simulink model "c00003M_harness"  (R2018a)
settings: Solver=FixedStepAuto  StartTime=0.0  StopTime=300  FixedStep=0.1  RelTol=1e-3
undefined symbols (not defined in the file): A1, hmax, PriorityTank, R1, R2, sigbuilder_block
(part 5 of 44)

== system c00003M_harness/M022 ==
  note: VALUES
      | ---------------------------------
      | ControlType = 1 | 2 | 3
      | FillTank = 0 | 1
      | EmptyTank = 0 | 1
      | ManualReference between 0 and 1
      | Tempreature between 0 and 100
      | EmergencyButton = 0 | 1
      | LiquidLevel between 0 and 1 (hmax)
  note: Inputs For Tank2
  note: NAMES
      | --------------------------------------------
      | CT1 = ControlType Tank 1
      | F1 = Fill Tank 1
      | E1 = Empty Tank 1
      | MR1 = Manual Reference Tank1
      | T1 = Temperature Tank 1
      | EB1 = Emergency Button Tank 1
      | LL1 = Liquid Level 1
  note: Inputs For Tank3
  note: Inputs For Tank1
  CT1 : Inport
  F1 : Inport  Port=2
  E1 : Inport  Port=3
  MR1 : Inport  Port=4
  T1 : Inport  Port=5
  EB1 : Inport  Port=6
  CT2 : Inport  Port=7
  F2 : Inport  Port=8
  E2 : Inport  Port=9
  MR2 : Inport  Port=10
  T2 : Inport  Port=11
  EB2 : Inport  Port=12
  Tank1 : Subsystem
  Tank2 : Subsystem
  LL1 : Outport
  LL2 : Outport  Port=2
  wires:
  EB1/1 -> Tank1/6(EB1)
  Tank2/1(LL2) -> LL2/1, Tank1/7(LL2)
  EB2/1 -> Tank2/6(EB2)
  CT2/1 -> Tank2/1(CT2)
  MR1/1 -> Tank1/4(MR1)
  T1/1 -> Tank1/5(T1)
  Tank1/1(LL1) -> LL1/1, Tank2/7(LL1)
  F2/1 -> Tank2/2(F2)
  E2/1 -> Tank2/3(E2)
  F1/1 -> Tank1/2(F1)
  E1/1 -> Tank1/3(E1)
  T2/1 -> Tank2/5(T2)
  CT1/1 -> Tank1/1(CT1)
  MR2/1 -> Tank2/4(MR2)

== system c00003M_harness/M023 ==
  note: VALUES
      | ---------------------------------
      | ControlType = 1 | 2 | 3
      | FillTank = 0 | 1
      | EmptyTank = 0 | 1
      | ManualReference between 0 and 1
      | Tempreature between 0 and 100
      | EmergencyButton = 0 | 1
      | LiquidLevel between 0 and 1 (hmax)
  note: Inputs For Tank2
  note: NAMES
      | --------------------------------------------
      | CT1 = ControlType Tank 1
      | F1 = Fill Tank 1
      | E1 = Empty Tank 1
      | MR1 = Manual Reference Tank1
      | T1 = Temperature Tank 1
      | EB1 = Emergency Button Tank 1
      | LL1 = Liquid Level 1
  note: Inputs For Tank3
  note: Inputs For Tank1
  CT1 : Inport
  F1 : Inport  Port=2
  E1 : Inport  Port=3
  MR1 : Inport  Port=4
  T1 : Inport  Port=5
  EB1 : Inport  Port=6
  CT2 : Inport  Port=7
  F2 : Inport  Port=8
  E2 : Inport  Port=9
  MR2 : Inport  Port=10
  T2 : Inport  Port=11
  EB2 : Inport  Port=12
  Tank1 : Subsystem
  Tank2 : Subsystem
  LL1 : Outport
  LL2 : Outport  Port=2
  wires:
  EB1/1 -> Tank1/6(EB1)
  Tank2/1(LL2) -> LL2/1, Tank1/7(LL2)
  EB2/1 -> Tank2/6(EB2)
  CT2/1 -> Tank2/1(CT2)
  MR1/1 -> Tank1/4(MR1)
  T1/1 -> Tank1/5(T1)
  Tank1/1(LL1) -> LL1/1, Tank2/7(LL1)
  F2/1 -> Tank2/2(F2)
  E2/1 -> Tank2/3(E2)
  F1/1 -> Tank1/2(F1)
  E1/1 -> Tank1/3(E1)
  T2/1 -> Tank2/5(T2)
  CT1/1 -> Tank1/1(CT1)
  MR2/1 -> Tank2/4(MR2)

== system c00003M_harness/M024 ==
  note: VALUES
      | ---------------------------------
      | ControlType = 1 | 2 | 3
      | FillTank = 0 | 1
      | EmptyTank = 0 | 1
      | ManualReference between 0 and 1
      | Tempreature between 0 and 100
      | EmergencyButton = 0 | 1
      | LiquidLevel between 0 and 1 (hmax)
  note: Inputs For Tank2
  note: NAMES
      | --------------------------------------------
      | CT1 = ControlType Tank 1
      | F1 = Fill Tank 1
      | E1 = Empty Tank 1
      | MR1 = Manual Reference Tank1
      | T1 = Temperature Tank 1
      | EB1 = Emergency Button Tank 1
      | LL1 = Liquid Level 1
  note: Inputs For Tank3
  note: Inputs For Tank1
  CT1 : Inport
  F1 : Inport  Port=2
  E1 : Inport  Port=3
  MR1 : Inport  Port=4
  T1 : Inport  Port=5
  EB1 : Inport  Port=6
  CT2 : Inport  Port=7
  F2 : Inport  Port=8
  E2 : Inport  Port=9
  MR2 : Inport  Port=10
  T2 : Inport  Port=11
  EB2 : Inport  Port=12
  Tank1 : Subsystem
  Tank2 : Subsystem
  LL1 : Outport
  LL2 : Outport  Port=2
  wires:
  EB1/1 -> Tank1/6(EB1)
  Tank2/1(LL2) -> LL2/1, Tank1/7(LL2)
  EB2/1 -> Tank2/6(EB2)
  CT2/1 -> Tank2/1(CT2)
  MR1/1 -> Tank1/4(MR1)
  T1/1 -> Tank1/5(T1)
  Tank1/1(LL1) -> LL1/1, Tank2/7(LL1)
  F2/1 -> Tank2/2(F2)
  E2/1 -> Tank2/3(E2)
  F1/1 -> Tank1/2(F1)
  E1/1 -> Tank1/3(E1)
  T2/1 -> Tank2/5(T2)
  CT1/1 -> Tank1/1(CT1)
  MR2/1 -> Tank2/4(MR2)

== system c00003M_harness/M025 ==
  note: VALUES
      | ---------------------------------
      | ControlType = 1 | 2 | 3
      | FillTank = 0 | 1
      | EmptyTank = 0 | 1
      | ManualReference between 0 and 1
      | Tempreature between 0 and 100
      | EmergencyButton = 0 | 1
      | LiquidLevel between 0 and 1 (hmax)
  note: Inputs For Tank2
  note: NAMES
      | --------------------------------------------
      | CT1 = ControlType Tank 1
      | F1 = Fill Tank 1
      | E1 = Empty Tank 1
      | MR1 = Manual Reference Tank1
      | T1 = Temperature Tank 1
      | EB1 = Emergency Button Tank 1
      | LL1 = Liquid Level 1
  note: Inputs For Tank3
  note: Inputs For Tank1
  CT1 : Inport
  F1 : Inport  Port=2
  E1 : Inport  Port=3
  MR1 : Inport  Port=4
  T1 : Inport  Port=5
  EB1 : Inport  Port=6
  CT2 : Inport  Port=7
  F2 : Inport  Port=8
  E2 : Inport  Port=9
  MR2 : Inport  Port=10
  T2 : Inport  Port=11
  EB2 : Inport  Port=12
  Tank1 : Subsystem
  Tank2 : Subsystem
  LL1 : Outport
  LL2 : Outport  Port=2
  wires:
  EB1/1 -> Tank1/6(EB1)
  Tank2/1(LL2) -> LL2/1, Tank1/7(LL2)
  EB2/1 -> Tank2/6(EB2)
  CT2/1 -> Tank2/1(CT2)
  MR1/1 -> Tank1/4(MR1)
  T1/1 -> Tank1/5(T1)
  Tank1/1(LL1) -> LL1/1, Tank2/7(LL1)
  F2/1 -> Tank2/2(F2)
  E2/1 -> Tank2/3(E2)
  F1/1 -> Tank1/2(F1)
  E1/1 -> Tank1/3(E1)
  T2/1 -> Tank2/5(T2)
  CT1/1 -> Tank1/1(CT1)
  MR2/1 -> Tank2/4(MR2)

== system c00003M_harness/M026 ==
  note: VALUES
      | ---------------------------------
      | ControlType = 1 | 2 | 3
      | FillTank = 0 | 1
      | EmptyTank = 0 | 1
      | ManualReference between 0 and 1
      | Tempreature between 0 and 100
      | EmergencyButton = 0 | 1
      | LiquidLevel between 0 and 1 (hmax)
  note: Inputs For Tank2
  note: NAMES
      | --------------------------------------------
      | CT1 = ControlType Tank 1
      | F1 = Fill Tank 1
      | E1 = Empty Tank 1
      | MR1 = Manual Reference Tank1
      | T1 = Temperature Tank 1
      | EB1 = Emergency Button Tank 1
      | LL1 = Liquid Level 1
  note: Inputs For Tank3
  note: Inputs For Tank1
  CT1 : Inport
  F1 : Inport  Port=2
  E1 : Inport  Port=3
  MR1 : Inport  Port=4
  T1 : Inport  Port=5
  EB1 : Inport  Port=6
  CT2 : Inport  Port=7
  F2 : Inport  Port=8
  E2 : Inport  Port=9
  MR2 : Inport  Port=10
  T2 : Inport  Port=11
  EB2 : Inport  Port=12
  Tank1 : Subsystem
  Tank2 : Subsystem
  LL1 : Outport
  LL2 : Outport  Port=2
  wires:
  EB1/1 -> Tank1/6(EB1)
  Tank2/1(LL2) -> LL2/1, Tank1/7(LL2)
  EB2/1 -> Tank2/6(EB2)
  CT2/1 -> Tank2/1(CT2)
  MR1/1 -> Tank1/4(MR1)
  T1/1 -> Tank1/5(T1)
  Tank1/1(LL1) -> LL1/1, Tank2/7(LL1)
  F2/1 -> Tank2/2(F2)
  E2/1 -> Tank2/3(E2)
  F1/1 -> Tank1/2(F1)
  E1/1 -> Tank1/3(E1)
  T2/1 -> Tank2/5(T2)
  CT1/1 -> Tank1/1(CT1)
  MR2/1 -> Tank2/4(MR2)

== system c00003M_harness/M027 ==
  note: VALUES
      | ---------------------------------
      | ControlType = 1 | 2 | 3
      | FillTank = 0 | 1
      | EmptyTank = 0 | 1
      | ManualReference between 0 and 1
      | Tempreature between 0 and 100
      | EmergencyButton = 0 | 1
      | LiquidLevel between 0 and 1 (hmax)
  note: Inputs For Tank2
  note: NAMES
      | --------------------------------------------
      | CT1 = ControlType Tank 1
      | F1 = Fill Tank 1
      | E1 = Empty Tank 1
      | MR1 = Manual Reference Tank1
      | T1 = Temperature Tank 1
      | EB1 = Emergency Button Tank 1
      | LL1 = Liquid Level 1
  note: Inputs For Tank3
  note: Inputs For Tank1
  CT1 : Inport
  F1 : Inport  Port=2
  E1 : Inport  Port=3
  MR1 : Inport  Port=4
  T1 : Inport  Port=5
  EB1 : Inport  Port=6
  CT2 : Inport  Port=7
  F2 : Inport  Port=8
  E2 : Inport  Port=9
  MR2 : Inport  Port=10
  T2 : Inport  Port=11
  EB2 : Inport  Port=12
  Tank1 : Subsystem
  Tank2 : Subsystem
  LL1 : Outport
  LL2 : Outport  Port=2
  wires:
  EB1/1 -> Tank1/6(EB1)
  Tank2/1(LL2) -> LL2/1, Tank1/7(LL2)
  EB2/1 -> Tank2/6(EB2)
  CT2/1 -> Tank2/1(CT2)
  MR1/1 -> Tank1/4(MR1)
  T1/1 -> Tank1/5(T1)
  Tank1/1(LL1) -> LL1/1, Tank2/7(LL1)
  F2/1 -> Tank2/2(F2)
  E2/1 -> Tank2/3(E2)
  F1/1 -> Tank1/2(F1)
  E1/1 -> Tank1/3(E1)
  T2/1 -> Tank2/5(T2)
  CT1/1 -> Tank1/1(CT1)
  MR2/1 -> Tank2/4(MR2)

== system c00003M_harness/M028 ==
  note: VALUES
      | ---------------------------------
      | ControlType = 1 | 2 | 3
      | FillTank = 0 | 1
      | EmptyTank = 0 | 1
      | ManualReference between 0 and 1
      | Tempreature between 0 and 100
      | EmergencyButton = 0 | 1
      | LiquidLevel between 0 and 1 (hmax)
  note: Inputs For Tank2
  note: NAMES
      | --------------------------------------------
      | CT1 = ControlType Tank 1
      | F1 = Fill Tank 1
      | E1 = Empty Tank 1
      | MR1 = Manual Reference Tank1
      | T1 = Temperature Tank 1
      | EB1 = Emergency Button Tank 1
      | LL1 = Liquid Level 1
  note: Inputs For Tank3
  note: Inputs For Tank1
  CT1 : Inport
  F1 : Inport  Port=2
  E1 : Inport  Port=3
  MR1 : Inport  Port=4
  T1 : Inport  Port=5
  EB1 : Inport  Port=6
  CT2 : Inport  Port=7
  F2 : Inport  Port=8
  E2 : Inport  Port=9
  MR2 : Inport  Port=10
  T2 : Inport  Port=11
  EB2 : Inport  Port=12
  Tank1 : Subsystem
  Tank2 : Subsystem
  LL1 : Outport
  LL2 : Outport  Port=2
  wires:
  EB1/1 -> Tank1/6(EB1)
  Tank2/1(LL2) -> LL2/1, Tank1/7(LL2)
  EB2/1 -> Tank2/6(EB2)
  CT2/1 -> Tank2/1(CT2)
  MR1/1 -> Tank1/4(MR1)
  T1/1 -> Tank1/5(T1)
  Tank1/1(LL1) -> LL1/1, Tank2/7(LL1)
  F2/1 -> Tank2/2(F2)
  E2/1 -> Tank2/3(E2)
  F1/1 -> Tank1/2(F1)
  E1/1 -> Tank1/3(E1)
  T2/1 -> Tank2/5(T2)
  CT1/1 -> Tank1/1(CT1)
  MR2/1 -> Tank2/4(MR2)

== system c00003M_harness/M029 ==
  note: VALUES
      | ---------------------------------
      | ControlType = 1 | 2 | 3
      | FillTank = 0 | 1
      | EmptyTank = 0 | 1
      | ManualReference between 0 and 1
      | Tempreature between 0 and 100
      | EmergencyButton = 0 | 1
      | LiquidLevel between 0 and 1 (hmax)
  note: Inputs For Tank2
  note: NAMES
      | --------------------------------------------
      | CT1 = ControlType Tank 1
      | F1 = Fill Tank 1
      | E1 = Empty Tank 1
      | MR1 = Manual Reference Tank1
      | T1 = Temperature Tank 1
      | EB1 = Emergency Button Tank 1
      | LL1 = Liquid Level 1
  note: Inputs For Tank3
  note: Inputs For Tank1
  CT1 : Inport
  F1 : Inport  Port=2
  E1 : Inport  Port=3
  MR1 : Inport  Port=4
  T1 : Inport  Port=5
  EB1 : Inport  Port=6
  CT2 : Inport  Port=7
  F2 : Inport  Port=8
  E2 : Inport  Port=9
  MR2 : Inport  Port=10
  T2 : Inport  Port=11
  EB2 : Inport  Port=12
  Tank1 : Subsystem
  Tank2 : Subsystem
  LL1 : Outport
  LL2 : Outport  Port=2
  wires:
  EB1/1 -> Tank1/6(EB1)
  Tank2/1(LL2) -> LL2/1, Tank1/7(LL2)
  EB2/1 -> Tank2/6(EB2)
  CT2/1 -> Tank2/1(CT2)
  MR1/1 -> Tank1/4(MR1)
  T1/1 -> Tank1/5(T1)
  Tank1/1(LL1) -> LL1/1, Tank2/7(LL1)
  F2/1 -> Tank2/2(F2)
  E2/1 -> Tank2/3(E2)
  F1/1 -> Tank1/2(F1)
  E1/1 -> Tank1/3(E1)
  T2/1 -> Tank2/5(T2)
  CT1/1 -> Tank1/1(CT1)
  MR2/1 -> Tank2/4(MR2)

== system c00003M_harness/M030 ==
  note: VALUES
      | ---------------------------------
      | ControlType = 1 | 2 | 3
      | FillTank = 0 | 1
      | EmptyTank = 0 | 1
      | ManualReference between 0 and 1
      | Tempreature between 0 and 100
      | EmergencyButton = 0 | 1
      | LiquidLevel between 0 and 1 (hmax)
  note: Inputs For Tank2
  note: NAMES
      | --------------------------------------------
      | CT1 = ControlType Tank 1
      | F1 = Fill Tank 1
      | E1 = Empty Tank 1
      | MR1 = Manual Reference Tank1
      | T1 = Temperature Tank 1
      | EB1 = Emergency Button Tank 1
      | LL1 = Liquid Level 1
  note: Inputs For Tank3
  note: Inputs For Tank1
  CT1 : Inport
  F1 : Inport  Port=2
  E1 : Inport  Port=3
  MR1 : Inport  Port=4
  T1 : Inport  Port=5
  EB1 : Inport  Port=6
  CT2 : Inport  Port=7
  F2 : Inport  Port=8
  E2 : Inport  Port=9
  MR2 : Inport  Port=10
  T2 : Inport  Port=11
  EB2 : Inport  Port=12
  Tank1 : Subsystem
  Tank2 : Subsystem
  LL1 : Outport
  LL2 : Outport  Port=2
  wires:
  EB1/1 -> Tank1/6(EB1)
  Tank2/1(LL2) -> LL2/1, Tank1/7(LL2)
  EB2/1 -> Tank2/6(EB2)
  CT2/1 -> Tank2/1(CT2)
  MR1/1 -> Tank1/4(MR1)
  T1/1 -> Tank1/5(T1)
  Tank1/1(LL1) -> LL1/1, Tank2/7(LL1)
  F2/1 -> Tank2/2(F2)
  E2/1 -> Tank2/3(E2)
  F1/1 -> Tank1/2(F1)
  E1/1 -> Tank1/3(E1)
  T2/1 -> Tank2/5(T2)
  CT1/1 -> Tank1/1(CT1)
  MR2/1 -> Tank2/4(MR2)

== system c00003M_harness/M031 ==
  note: VALUES
      | ---------------------------------
      | ControlType = 1 | 2 | 3
      | FillTank = 0 | 1
      | EmptyTank = 0 | 1
      | ManualReference between 0 and 1
      | Tempreature between 0 and 100
      | EmergencyButton = 0 | 1
      | LiquidLevel between 0 and 1 (hmax)
  note: Inputs For Tank2
  note: NAMES
      | --------------------------------------------
      | CT1 = ControlType Tank 1
      | F1 = Fill Tank 1
      | E1 = Empty Tank 1
      | MR1 = Manual Reference Tank1
      | T1 = Temperature Tank 1
      | EB1 = Emergency Button Tank 1
      | LL1 = Liquid Level 1
  note: Inputs For Tank3
  note: Inputs For Tank1
  CT1 : Inport
  F1 : Inport  Port=2
  E1 : Inport  Port=3
  MR1 : Inport  Port=4
  T1 : Inport  Port=5
  EB1 : Inport  Port=6
  CT2 : Inport  Port=7
  F2 : Inport  Port=8
  E2 : Inport  Port=9
  MR2 : Inport  Port=10
  T2 : Inport  Port=11
  EB2 : Inport  Port=12
  Tank1 : Subsystem
  Tank2 : Subsystem
  LL1 : Outport
  LL2 : Outport  Port=2
  wires:
  EB1/1 -> Tank1/6(EB1)
  Tank2/1(LL2) -> LL2/1, Tank1/7(LL2)
  EB2/1 -> Tank2/6(EB2)
  CT2/1 -> Tank2/1(CT2)
  MR1/1 -> Tank1/4(MR1)
  T1/1 -> Tank1/5(T1)
  Tank1/1(LL1) -> LL1/1, Tank2/7(LL1)
  F2/1 -> Tank2/2(F2)
  E2/1 -> Tank2/3(E2)
  F1/1 -> Tank1/2(F1)
  E1/1 -> Tank1/3(E1)
  T2/1 -> Tank2/5(T2)
  CT1/1 -> Tank1/1(CT1)
  MR2/1 -> Tank2/4(MR2)

== system c00003M_harness/M032 ==
  note: VALUES
      | ---------------------------------
      | ControlType = 1 | 2 | 3
      | FillTank = 0 | 1
      | EmptyTank = 0 | 1
      | ManualReference between 0 and 1
      | Tempreature between 0 and 100
      | EmergencyButton = 0 | 1
      | LiquidLevel between 0 and 1 (hmax)
  note: Inputs For Tank2
  note: NAMES
      | --------------------------------------------
      | CT1 = ControlType Tank 1
      | F1 = Fill Tank 1
      | E1 = Empty Tank 1
      | MR1 = Manual Reference Tank1
      | T1 = Temperature Tank 1
      | EB1 = Emergency Button Tank 1
      | LL1 = Liquid Level 1
  note: Inputs For Tank3
  note: Inputs For Tank1
  CT1 : Inport
  F1 : Inport  Port=2
  E1 : Inport  Port=3
  MR1 : Inport  Port=4
  T1 : Inport  Port=5
  EB1 : Inport  Port=6
  CT2 : Inport  Port=7
  F2 : Inport  Port=8
  E2 : Inport  Port=9
  MR2 : Inport  Port=10
  T2 : Inport  Port=11
  EB2 : Inport  Port=12
  Tank1 : Subsystem
  Tank2 : Subsystem
  LL1 : Outport
  LL2 : Outport  Port=2
  wires:
  EB1/1 -> Tank1/6(EB1)
  Tank2/1(LL2) -> LL2/1, Tank1/7(LL2)
  EB2/1 -> Tank2/6(EB2)
  CT2/1 -> Tank2/1(CT2)
  MR1/1 -> Tank1/4(MR1)
  T1/1 -> Tank1/5(T1)
  Tank1/1(LL1) -> LL1/1, Tank2/7(LL1)
  F2/1 -> Tank2/2(F2)
  E2/1 -> Tank2/3(E2)
  F1/1 -> Tank1/2(F1)
  E1/1 -> Tank1/3(E1)
  T2/1 -> Tank2/5(T2)
  CT1/1 -> Tank1/1(CT1)
  MR2/1 -> Tank2/4(MR2)

== system c00003M_harness/M033 ==
  note: VALUES
      | ---------------------------------
      | ControlType = 1 | 2 | 3
      | FillTank = 0 | 1
      | EmptyTank = 0 | 1
      | ManualReference between 0 and 1
      | Tempreature between 0 and 100
      | EmergencyButton = 0 | 1
      | LiquidLevel between 0 and 1 (hmax)
  note: Inputs For Tank2
  note: NAMES
      | --------------------------------------------
      | CT1 = ControlType Tank 1
      | F1 = Fill Tank 1
      | E1 = Empty Tank 1
      | MR1 = Manual Reference Tank1
      | T1 = Temperature Tank 1
      | EB1 = Emergency Button Tank 1
      | LL1 = Liquid Level 1
  note: Inputs For Tank3
  note: Inputs For Tank1
  CT1 : Inport
  F1 : Inport  Port=2
  E1 : Inport  Port=3
  MR1 : Inport  Port=4
  T1 : Inport  Port=5
  EB1 : Inport  Port=6
  CT2 : Inport  Port=7
  F2 : Inport  Port=8
  E2 : Inport  Port=9
  MR2 : Inport  Port=10
  T2 : Inport  Port=11
  EB2 : Inport  Port=12
  Tank1 : Subsystem
  Tank2 : Subsystem
  LL1 : Outport
  LL2 : Outport  Port=2
  wires:
  EB1/1 -> Tank1/6(EB1)
  Tank2/1(LL2) -> LL2/1, Tank1/7(LL2)
  EB2/1 -> Tank2/6(EB2)
  CT2/1 -> Tank2/1(CT2)
  MR1/1 -> Tank1/4(MR1)
  T1/1 -> Tank1/5(T1)
  Tank1/1(LL1) -> LL1/1, Tank2/7(LL1)
  F2/1 -> Tank2/2(F2)
  E2/1 -> Tank2/3(E2)
  F1/1 -> Tank1/2(F1)
  E1/1 -> Tank1/3(E1)
  T2/1 -> Tank2/5(T2)
  CT1/1 -> Tank1/1(CT1)
  MR2/1 -> Tank2/4(MR2)

== system c00003M_harness/M034 ==
  note: VALUES
      | ---------------------------------
      | ControlType = 1 | 2 | 3
      | FillTank = 0 | 1
      | EmptyTank = 0 | 1
      | ManualReference between 0 and 1
      | Tempreature between 0 and 100
      | EmergencyButton = 0 | 1
      | LiquidLevel between 0 and 1 (hmax)
  note: Inputs For Tank2
  note: NAMES
      | --------------------------------------------
      | CT1 = ControlType Tank 1
      | F1 = Fill Tank 1
      | E1 = Empty Tank 1
      | MR1 = Manual Reference Tank1
      | T1 = Temperature Tank 1
      | EB1 = Emergency Button Tank 1
      | LL1 = Liquid Level 1
  note: Inputs For Tank3
  note: Inputs For Tank1
  CT1 : Inport
  F1 : Inport  Port=2
  E1 : Inport  Port=3
  MR1 : Inport  Port=4
  T1 : Inport  Port=5
  EB1 : Inport  Port=6
  CT2 : Inport  Port=7
  F2 : Inport  Port=8
  E2 : Inport  Port=9
  MR2 : Inport  Port=10
  T2 : Inport  Port=11
  EB2 : Inport  Port=12
  Tank1 : Subsystem
  Tank2 : Subsystem
  LL1 : Outport
  LL2 : Outport  Port=2
  wires:
  EB1/1 -> Tank1/6(EB1)
  Tank2/1(LL2) -> LL2/1, Tank1/7(LL2)
  EB2/1 -> Tank2/6(EB2)
  CT2/1 -> Tank2/1(CT2)
  MR1/1 -> Tank1/4(MR1)
  T1/1 -> Tank1/5(T1)
  Tank1/1(LL1) -> LL1/1, Tank2/7(LL1)
  F2/1 -> Tank2/2(F2)
  E2/1 -> Tank2/3(E2)
  F1/1 -> Tank1/2(F1)
  E1/1 -> Tank1/3(E1)
  T2/1 -> Tank2/5(T2)
  CT1/1 -> Tank1/1(CT1)
  MR2/1 -> Tank2/4(MR2)

== system c00003M_harness/M035 ==
  note: VALUES
      | ---------------------------------
      | ControlType = 1 | 2 | 3
      | FillTank = 0 | 1
      | EmptyTank = 0 | 1
      | ManualReference between 0 and 1
      | Tempreature between 0 and 100
      | EmergencyButton = 0 | 1
      | LiquidLevel between 0 and 1 (hmax)
  note: Inputs For Tank2
  note: NAMES
      | --------------------------------------------
      | CT1 = ControlType Tank 1
      | F1 = Fill Tank 1
      | E1 = Empty Tank 1
      | MR1 = Manual Reference Tank1
      | T1 = Temperature Tank 1
      | EB1 = Emergency Button Tank 1
      | LL1 = Liquid Level 1
  note: Inputs For Tank3
  note: Inputs For Tank1
  CT1 : Inport
  F1 : Inport  Port=2
  E1 : Inport  Port=3
  MR1 : Inport  Port=4
  T1 : Inport  Port=5
  EB1 : Inport  Port=6
  CT2 : Inport  Port=7
  F2 : Inport  Port=8
  E2 : Inport  Port=9
  MR2 : Inport  Port=10
  T2 : Inport  Port=11
  EB2 : Inport  Port=12
  Tank1 : Subsystem
  Tank2 : Subsystem
  LL1 : Outport
  LL2 : Outport  Port=2
  wires:
  EB1/1 -> Tank1/6(EB1)
  Tank2/1(LL2) -> LL2/1, Tank1/7(LL2)
  EB2/1 -> Tank2/6(EB2)
  CT2/1 -> Tank2/1(CT2)
  MR1/1 -> Tank1/4(MR1)
  T1/1 -> Tank1/5(T1)
  Tank1/1(LL1) -> LL1/1, Tank2/7(LL1)
  F2/1 -> Tank2/2(F2)
  E2/1 -> Tank2/3(E2)
  F1/1 -> Tank1/2(F1)
  E1/1 -> Tank1/3(E1)
  T2/1 -> Tank2/5(T2)
  CT1/1 -> Tank1/1(CT1)
  MR2/1 -> Tank2/4(MR2)

== system c00003M_harness/M036 ==
  note: VALUES
      | ---------------------------------
      | ControlType = 1 | 2 | 3
      | FillTank = 0 | 1
      | EmptyTank = 0 | 1
      | ManualReference between 0 and 1
      | Tempreature between 0 and 100
      | EmergencyButton = 0 | 1
      | LiquidLevel between 0 and 1 (hmax)
  note: Inputs For Tank2
  note: NAMES
      | --------------------------------------------
      | CT1 = ControlType Tank 1
      | F1 = Fill Tank 1
      | E1 = Empty Tank 1
      | MR1 = Manual Reference Tank1
      | T1 = Temperature Tank 1
      | EB1 = Emergency Button Tank 1
      | LL1 = Liquid Level 1
  note: Inputs For Tank3
  note: Inputs For Tank1
  CT1 : Inport
  F1 : Inport  Port=2
  E1 : Inport  Port=3
  MR1 : Inport  Port=4
  T1 : Inport  Port=5
  EB1 : Inport  Port=6
  CT2 : Inport  Port=7
  F2 : Inport  Port=8
  E2 : Inport  Port=9
  MR2 : Inport  Port=10
  T2 : Inport  Port=11
  EB2 : Inport  Port=12
  Tank1 : Subsystem
  Tank2 : Subsystem
  LL1 : Outport
  LL2 : Outport  Port=2
  wires:
  EB1/1 -> Tank1/6(EB1)
  Tank2/1(LL2) -> LL2/1, Tank1/7(LL2)
  EB2/1 -> Tank2/6(EB2)
  CT2/1 -> Tank2/1(CT2)
  MR1/1 -> Tank1/4(MR1)
  T1/1 -> Tank1/5(T1)
  Tank1/1(LL1) -> LL1/1, Tank2/7(LL1)
  F2/1 -> Tank2/2(F2)
  E2/1 -> Tank2/3(E2)
  F1/1 -> Tank1/2(F1)
  E1/1 -> Tank1/3(E1)
  T2/1 -> Tank2/5(T2)
  CT1/1 -> Tank1/1(CT1)
  MR2/1 -> Tank2/4(MR2)

== system c00003M_harness/M037 ==
  note: VALUES
      | ---------------------------------
      | ControlType = 1 | 2 | 3
      | FillTank = 0 | 1
      | EmptyTank = 0 | 1
      | ManualReference between 0 and 1
      | Tempreature between 0 and 100
      | EmergencyButton = 0 | 1
      | LiquidLevel between 0 and 1 (hmax)
  note: Inputs For Tank2
  note: NAMES
      | --------------------------------------------
      | CT1 = ControlType Tank 1
      | F1 = Fill Tank 1
      | E1 = Empty Tank 1
      | MR1 = Manual Reference Tank1
      | T1 = Temperature Tank 1
      | EB1 = Emergency Button Tank 1
      | LL1 = Liquid Level 1
  note: Inputs For Tank3
  note: Inputs For Tank1
  CT1 : Inport
  F1 : Inport  Port=2
  E1 : Inport  Port=3
  MR1 : Inport  Port=4
  T1 : Inport  Port=5
  EB1 : Inport  Port=6
  CT2 : Inport  Port=7
  F2 : Inport  Port=8
  E2 : Inport  Port=9
  MR2 : Inport  Port=10
  T2 : Inport  Port=11
  EB2 : Inport  Port=12
  Tank1 : Subsystem
  Tank2 : Subsystem
  LL1 : Outport
  LL2 : Outport  Port=2
  wires:
  EB1/1 -> Tank1/6(EB1)
  Tank2/1(LL2) -> LL2/1, Tank1/7(LL2)
  EB2/1 -> Tank2/6(EB2)
  CT2/1 -> Tank2/1(CT2)
  MR1/1 -> Tank1/4(MR1)
  T1/1 -> Tank1/5(T1)
  Tank1/1(LL1) -> LL1/1, Tank2/7(LL1)
  F2/1 -> Tank2/2(F2)
  E2/1 -> Tank2/3(E2)
  F1/1 -> Tank1/2(F1)
  E1/1 -> Tank1/3(E1)
  T2/1 -> Tank2/5(T2)
  CT1/1 -> Tank1/1(CT1)
  MR2/1 -> Tank2/4(MR2)

== system c00003M_harness/M038 ==
  note: VALUES
      | ---------------------------------
      | ControlType = 1 | 2 | 3
      | FillTank = 0 | 1
      | EmptyTank = 0 | 1
      | ManualReference between 0 and 1
      | Tempreature between 0 and 100
      | EmergencyButton = 0 | 1
      | LiquidLevel between 0 and 1 (hmax)
  note: Inputs For Tank2
  note: NAMES
      | --------------------------------------------
      | CT1 = ControlType Tank 1
      | F1 = Fill Tank 1
      | E1 = Empty Tank 1
      | MR1 = Manual Reference Tank1
      | T1 = Temperature Tank 1
      | EB1 = Emergency Button Tank 1
      | LL1 = Liquid Level 1
  note: Inputs For Tank3
  note: Inputs For Tank1
  CT1 : Inport
  F1 : Inport  Port=2
  E1 : Inport  Port=3
  MR1 : Inport  Port=4
  T1 : Inport  Port=5
  EB1 : Inport  Port=6
  CT2 : Inport  Port=7
  F2 : Inport  Port=8
  E2 : Inport  Port=9
  MR2 : Inport  Port=10
  T2 : Inport  Port=11
  EB2 : Inport  Port=12
  Tank1 : Subsystem
  Tank2 : Subsystem
  LL1 : Outport
  LL2 : Outport  Port=2
  wires:
  EB1/1 -> Tank1/6(EB1)
  Tank2/1(LL2) -> LL2/1, Tank1/7(LL2)
  EB2/1 -> Tank2/6(EB2)
  CT2/1 -> Tank2/1(CT2)
  MR1/1 -> Tank1/4(MR1)
  T1/1 -> Tank1/5(T1)
  Tank1/1(LL1) -> LL1/1, Tank2/7(LL1)
  F2/1 -> Tank2/2(F2)
  E2/1 -> Tank2/3(E2)
  F1/1 -> Tank1/2(F1)
  E1/1 -> Tank1/3(E1)
  T2/1 -> Tank2/5(T2)
  CT1/1 -> Tank1/1(CT1)
  MR2/1 -> Tank2/4(MR2)

== system c00003M_harness/M039 ==
  note: VALUES
      | ---------------------------------
      | ControlType = 1 | 2 | 3
      | FillTank = 0 | 1
      | EmptyTank = 0 | 1
      | ManualReference between 0 and 1
      | Tempreature between 0 and 100
      | EmergencyButton = 0 | 1
      | LiquidLevel between 0 and 1 (hmax)
  note: Inputs For Tank2
  note: NAMES
      | --------------------------------------------
      | CT1 = ControlType Tank 1
      | F1 = Fill Tank 1
      | E1 = Empty Tank 1
      | MR1 = Manual Reference Tank1
      | T1 = Temperature Tank 1
      | EB1 = Emergency Button Tank 1
      | LL1 = Liquid Level 1
  note: Inputs For Tank3
  note: Inputs For Tank1
  CT1 : Inport
  F1 : Inport  Port=2
  E1 : Inport  Port=3
  MR1 : Inport  Port=4
  T1 : Inport  Port=5
  EB1 : Inport  Port=6
  CT2 : Inport  Port=7
  F2 : Inport  Port=8
  E2 : Inport  Port=9
  MR2 : Inport  Port=10
  T2 : Inport  Port=11
  EB2 : Inport  Port=12
  Tank1 : Subsystem
  Tank2 : Subsystem
  LL1 : Outport
  LL2 : Outport  Port=2
  wires:
  EB1/1 -> Tank1/6(EB1)
  Tank2/1(LL2) -> LL2/1, Tank1/7(LL2)
  EB2/1 -> Tank2/6(EB2)
  CT2/1 -> Tank2/1(CT2)
  MR1/1 -> Tank1/4(MR1)
  T1/1 -> Tank1/5(T1)
  Tank1/1(LL1) -> LL1/1, Tank2/7(LL1)
  F2/1 -> Tank2/2(F2)
  E2/1 -> Tank2/3(E2)
  F1/1 -> Tank1/2(F1)
  E1/1 -> Tank1/3(E1)
  T2/1 -> Tank2/5(T2)
  CT1/1 -> Tank1/1(CT1)
  MR2/1 -> Tank2/4(MR2)

== system c00003M_harness/M040 ==
  note: VALUES
      | ---------------------------------
      | ControlType = 1 | 2 | 3
      | FillTank = 0 | 1
      | EmptyTank = 0 | 1
      | ManualReference between 0 and 1
      | Tempreature between 0 and 100
      | EmergencyButton = 0 | 1
      | LiquidLevel between 0 and 1 (hmax)
  note: Inputs For Tank2
  note: NAMES
      | --------------------------------------------
      | CT1 = ControlType Tank 1
      | F1 = Fill Tank 1
      | E1 = Empty Tank 1
      | MR1 = Manual Reference Tank1
      | T1 = Temperature Tank 1
      | EB1 = Emergency Button Tank 1
      | LL1 = Liquid Level 1
  note: Inputs For Tank3
  note: Inputs For Tank1
  CT1 : Inport
  F1 : Inport  Port=2
  E1 : Inport  Port=3
  MR1 : Inport  Port=4
  T1 : Inport  Port=5
  EB1 : Inport  Port=6
  CT2 : Inport  Port=7
  F2 : Inport  Port=8
  E2 : Inport  Port=9
  MR2 : Inport  Port=10
  T2 : Inport  Port=11
  EB2 : Inport  Port=12
  Tank1 : Subsystem
  Tank2 : Subsystem
  LL1 : Outport
  LL2 : Outport  Port=2
  wires:
  EB1/1 -> Tank1/6(EB1)
  Tank2/1(LL2) -> LL2/1, Tank1/7(LL2)
  EB2/1 -> Tank2/6(EB2)
  CT2/1 -> Tank2/1(CT2)
  MR1/1 -> Tank1/4(MR1)
  T1/1 -> Tank1/5(T1)
  Tank1/1(LL1) -> LL1/1, Tank2/7(LL1)
  F2/1 -> Tank2/2(F2)
  E2/1 -> Tank2/3(E2)
  F1/1 -> Tank1/2(F1)
  E1/1 -> Tank1/3(E1)
  T2/1 -> Tank2/5(T2)
  CT1/1 -> Tank1/1(CT1)
  MR2/1 -> Tank2/4(MR2)

== system c00003M_harness/M041 ==
  note: VALUES
      | ---------------------------------
      | ControlType = 1 | 2 | 3
      | FillTank = 0 | 1
      | EmptyTank = 0 | 1
      | ManualReference between 0 and 1
      | Tempreature between 0 and 100
      | EmergencyButton = 0 | 1
      | LiquidLevel between 0 and 1 (hmax)
  note: Inputs For Tank2
  note: NAMES
      | --------------------------------------------
      | CT1 = ControlType Tank 1
      | F1 = Fill Tank 1
      | E1 = Empty Tank 1
      | MR1 = Manual Reference Tank1
      | T1 = Temperature Tank 1
      | EB1 = Emergency Button Tank 1
      | LL1 = Liquid Level 1
  note: Inputs For Tank3
  note: Inputs For Tank1
  CT1 : Inport
  F1 : Inport  Port=2
  E1 : Inport  Port=3
  MR1 : Inport  Port=4
  T1 : Inport  Port=5
  EB1 : Inport  Port=6
  CT2 : Inport  Port=7
  F2 : Inport  Port=8
  E2 : Inport  Port=9
  MR2 : Inport  Port=10
  T2 : Inport  Port=11
  EB2 : Inport  Port=12
  Tank1 : Subsystem
  Tank2 : Subsystem
  LL1 : Outport
  LL2 : Outport  Port=2
  wires:
  EB1/1 -> Tank1/6(EB1)
  Tank2/1(LL2) -> LL2/1, Tank1/7(LL2)
  EB2/1 -> Tank2/6(EB2)
  CT2/1 -> Tank2/1(CT2)
  MR1/1 -> Tank1/4(MR1)
  T1/1 -> Tank1/5(T1)
  Tank1/1(LL1) -> LL1/1, Tank2/7(LL1)
  F2/1 -> Tank2/2(F2)
  E2/1 -> Tank2/3(E2)
  F1/1 -> Tank1/2(F1)
  E1/1 -> Tank1/3(E1)
  T2/1 -> Tank2/5(T2)
  CT1/1 -> Tank1/1(CT1)
  MR2/1 -> Tank2/4(MR2)

== system c00003M_harness/M042 ==
  note: VALUES
      | ---------------------------------
      | ControlType = 1 | 2 | 3
      | FillTank = 0 | 1
      | EmptyTank = 0 | 1
      | ManualReference between 0 and 1
      | Tempreature between 0 and 100
      | EmergencyButton = 0 | 1
      | LiquidLevel between 0 and 1 (hmax)
  note: Inputs For Tank2
  note: NAMES
      | --------------------------------------------
      | CT1 = ControlType Tank 1
      | F1 = Fill Tank 1
      | E1 = Empty Tank 1
      | MR1 = Manual Reference Tank1
      | T1 = Temperature Tank 1
      | EB1 = Emergency Button Tank 1
      | LL1 = Liquid Level 1
  note: Inputs For Tank3
  note: Inputs For Tank1
  CT1 : Inport
  F1 : Inport  Port=2
  E1 : Inport  Port=3
  MR1 : Inport  Port=4
  T1 : Inport  Port=5
  EB1 : Inport  Port=6
  CT2 : Inport  Port=7
  F2 : Inport  Port=8
  E2 : Inport  Port=9
  MR2 : Inport  Port=10
  T2 : Inport  Port=11
  EB2 : Inport  Port=12
  Tank1 : Subsystem
  Tank2 : Subsystem
  LL1 : Outport
  LL2 : Outport  Port=2
  wires:
  EB1/1 -> Tank1/6(EB1)
  Tank2/1(LL2) -> LL2/1, Tank1/7(LL2)
  EB2/1 -> Tank2/6(EB2)
  CT2/1 -> Tank2/1(CT2)
  MR1/1 -> Tank1/4(MR1)
  T1/1 -> Tank1/5(T1)
  Tank1/1(LL1) -> LL1/1, Tank2/7(LL1)
  F2/1 -> Tank2/2(F2)
  E2/1 -> Tank2/3(E2)
  F1/1 -> Tank1/2(F1)
  E1/1 -> Tank1/3(E1)
  T2/1 -> Tank2/5(T2)
  CT1/1 -> Tank1/1(CT1)
  MR2/1 -> Tank2/4(MR2)

== system c00003M_harness/M043 ==
  note: VALUES
      | ---------------------------------
      | ControlType = 1 | 2 | 3
      | FillTank = 0 | 1
      | EmptyTank = 0 | 1
      | ManualReference between 0 and 1
      | Tempreature between 0 and 100
      | EmergencyButton = 0 | 1
      | LiquidLevel between 0 and 1 (hmax)
  note: Inputs For Tank2
  note: NAMES
      | --------------------------------------------
      | CT1 = ControlType Tank 1
      | F1 = Fill Tank 1
      | E1 = Empty Tank 1
      | MR1 = Manual Reference Tank1
      | T1 = Temperature Tank 1
      | EB1 = Emergency Button Tank 1
      | LL1 = Liquid Level 1
  note: Inputs For Tank3
  note: Inputs For Tank1
  CT1 : Inport
  F1 : Inport  Port=2
  E1 : Inport  Port=3
  MR1 : Inport  Port=4
  T1 : Inport  Port=5
  EB1 : Inport  Port=6
  CT2 : Inport  Port=7
  F2 : Inport  Port=8
  E2 : Inport  Port=9
  MR2 : Inport  Port=10
  T2 : Inport  Port=11
  EB2 : Inport  Port=12
  Tank1 : Subsystem
  Tank2 : Subsystem
  LL1 : Outport
  LL2 : Outport  Port=2
  wires:
  EB1/1 -> Tank1/6(EB1)
  Tank2/1(LL2) -> LL2/1, Tank1/7(LL2)
  EB2/1 -> Tank2/6(EB2)
  CT2/1 -> Tank2/1(CT2)
  MR1/1 -> Tank1/4(MR1)
  T1/1 -> Tank1/5(T1)
  Tank1/1(LL1) -> LL1/1, Tank2/7(LL1)
  F2/1 -> Tank2/2(F2)
  E2/1 -> Tank2/3(E2)
  F1/1 -> Tank1/2(F1)
  E1/1 -> Tank1/3(E1)
  T2/1 -> Tank2/5(T2)
  CT1/1 -> Tank1/1(CT1)
  MR2/1 -> Tank2/4(MR2)

== system c00003M_harness/M044 ==
  note: VALUES
      | ---------------------------------
      | ControlType = 1 | 2 | 3
      | FillTank = 0 | 1
      | EmptyTank = 0 | 1
      | ManualReference between 0 and 1
      | Tempreature between 0 and 100
      | EmergencyButton = 0 | 1
      | LiquidLevel between 0 and 1 (hmax)
  note: Inputs For Tank2
  note: NAMES
      | --------------------------------------------
      | CT1 = ControlType Tank 1
      | F1 = Fill Tank 1
      | E1 = Empty Tank 1
      | MR1 = Manual Reference Tank1
      | T1 = Temperature Tank 1
      | EB1 = Emergency Button Tank 1
      | LL1 = Liquid Level 1
  note: Inputs For Tank3
  note: Inputs For Tank1
  CT1 : Inport
  F1 : Inport  Port=2
  E1 : Inport  Port=3
  MR1 : Inport  Port=4
  T1 : Inport  Port=5
  EB1 : Inport  Port=6
  CT2 : Inport  Port=7
  F2 : Inport  Port=8
  E2 : Inport  Port=9
  MR2 : Inport  Port=10
  T2 : Inport  Port=11
  EB2 : Inport  Port=12
  Tank1 : Subsystem
  Tank2 : Subsystem
  LL1 : Outport
  LL2 : Outport  Port=2
  wires:
  EB1/1 -> Tank1/6(EB1)
  Tank2/1(LL2) -> LL2/1, Tank1/7(LL2)
  EB2/1 -> Tank2/6(EB2)
  CT2/1 -> Tank2/1(CT2)
  MR1/1 -> Tank1/4(MR1)
  T1/1 -> Tank1/5(T1)
  Tank1/1(LL1) -> LL1/1, Tank2/7(LL1)
  F2/1 -> Tank2/2(F2)
  E2/1 -> Tank2/3(E2)
  F1/1 -> Tank1/2(F1)
  E1/1 -> Tank1/3(E1)
  T2/1 -> Tank2/5(T2)
  CT1/1 -> Tank1/1(CT1)
  MR2/1 -> Tank2/4(MR2)

== system c00003M_harness/M045 ==
  note: VALUES
      | ---------------------------------
      | ControlType = 1 | 2 | 3
      | FillTank = 0 | 1
      | EmptyTank = 0 | 1
      | ManualReference between 0 and 1
      | Tempreature between 0 and 100
      | EmergencyButton = 0 | 1
      | LiquidLevel between 0 and 1 (hmax)
  note: Inputs For Tank2
  note: NAMES
      | --------------------------------------------
      | CT1 = ControlType Tank 1
      | F1 = Fill Tank 1
      | E1 = Empty Tank 1
      | MR1 = Manual Reference Tank1
      | T1 = Temperature Tank 1
      | EB1 = Emergency Button Tank 1
      | LL1 = Liquid Level 1
  note: Inputs For Tank3
  note: Inputs For Tank1
  CT1 : Inport
  F1 : Inport  Port=2
  E1 : Inport  Port=3
  MR1 : Inport  Port=4
  T1 : Inport  Port=5
  EB1 : Inport  Port=6
  CT2 : Inport  Port=7
  F2 : Inport  Port=8
  E2 : Inport  Port=9
  MR2 : Inport  Port=10
  T2 : Inport  Port=11
  EB2 : Inport  Port=12
  Tank1 : Subsystem
  Tank2 : Subsystem
  LL1 : Outport
  LL2 : Outport  Port=2
  wires:
  EB1/1 -> Tank1/6(EB1)
  Tank2/1(LL2) -> LL2/1, Tank1/7(LL2)
  EB2/1 -> Tank2/6(EB2)
  CT2/1 -> Tank2/1(CT2)
  MR1/1 -> Tank1/4(MR1)
  T1/1 -> Tank1/5(T1)
  Tank1/1(LL1) -> LL1/1, Tank2/7(LL1)
  F2/1 -> Tank2/2(F2)
  E2/1 -> Tank2/3(E2)
  F1/1 -> Tank1/2(F1)
  E1/1 -> Tank1/3(E1)
  T2/1 -> Tank2/5(T2)
  CT1/1 -> Tank1/1(CT1)
  MR2/1 -> Tank2/4(MR2)

== system c00003M_harness/M046 ==
  note: VALUES
      | ---------------------------------
      | ControlType = 1 | 2 | 3
      | FillTank = 0 | 1
      | EmptyTank = 0 | 1
      | ManualReference between 0 and 1
      | Tempreature between 0 and 100
      | EmergencyButton = 0 | 1
      | LiquidLevel between 0 and 1 (hmax)
  note: Inputs For Tank2
  note: NAMES
      | --------------------------------------------
      | CT1 = ControlType Tank 1
      | F1 = Fill Tank 1
      | E1 = Empty Tank 1
      | MR1 = Manual Reference Tank1
      | T1 = Temperature Tank 1
      | EB1 = Emergency Button Tank 1
      | LL1 = Liquid Level 1
  note: Inputs For Tank3
  note: Inputs For Tank1
  CT1 : Inport
  F1 : Inport  Port=2
  E1 : Inport  Port=3
  MR1 : Inport  Port=4
  T1 : Inport  Port=5
  EB1 : Inport  Port=6
  CT2 : Inport  Port=7
  F2 : Inport  Port=8
  E2 : Inport  Port=9
  MR2 : Inport  Port=10
  T2 : Inport  Port=11
  EB2 : Inport  Port=12
  Tank1 : Subsystem
  Tank2 : Subsystem
  LL1 : Outport
  LL2 : Outport  Port=2
  wires:
  EB1/1 -> Tank1/6(EB1)
  Tank2/1(LL2) -> LL2/1, Tank1/7(LL2)
  EB2/1 -> Tank2/6(EB2)
  CT2/1 -> Tank2/1(CT2)
  MR1/1 -> Tank1/4(MR1)
  T1/1 -> Tank1/5(T1)
  Tank1/1(LL1) -> LL1/1, Tank2/7(LL1)
  F2/1 -> Tank2/2(F2)
  E2/1 -> Tank2/3(E2)
  F1/1 -> Tank1/2(F1)
  E1/1 -> Tank1/3(E1)
  T2/1 -> Tank2/5(T2)
  CT1/1 -> Tank1/1(CT1)
  MR2/1 -> Tank2/4(MR2)

== system c00003M_harness/M047 ==
  note: VALUES
      | ---------------------------------
      | ControlType = 1 | 2 | 3
      | FillTank = 0 | 1
      | EmptyTank = 0 | 1
      | ManualReference between 0 and 1
      | Tempreature between 0 and 100
      | EmergencyButton = 0 | 1
      | LiquidLevel between 0 and 1 (hmax)
  note: Inputs For Tank2
  note: NAMES
      | --------------------------------------------
      | CT1 = ControlType Tank 1
      | F1 = Fill Tank 1
      | E1 = Empty Tank 1
      | MR1 = Manual Reference Tank1
      | T1 = Temperature Tank 1
      | EB1 = Emergency Button Tank 1
      | LL1 = Liquid Level 1
  note: Inputs For Tank3
  note: Inputs For Tank1
  CT1 : Inport
  F1 : Inport  Port=2
  E1 : Inport  Port=3
  MR1 : Inport  Port=4
  T1 : Inport  Port=5
  EB1 : Inport  Port=6
  CT2 : Inport  Port=7
  F2 : Inport  Port=8
  E2 : Inport  Port=9
  MR2 : Inport  Port=10
  T2 : Inport  Port=11
  EB2 : Inport  Port=12
  Tank1 : Subsystem
  Tank2 : Subsystem
  LL1 : Outport
  LL2 : Outport  Port=2
  wires:
  EB1/1 -> Tank1/6(EB1)
  Tank2/1(LL2) -> LL2/1, Tank1/7(LL2)
  EB2/1 -> Tank2/6(EB2)
  CT2/1 -> Tank2/1(CT2)
  MR1/1 -> Tank1/4(MR1)
  T1/1 -> Tank1/5(T1)
  Tank1/1(LL1) -> LL1/1, Tank2/7(LL1)
  F2/1 -> Tank2/2(F2)
  E2/1 -> Tank2/3(E2)
  F1/1 -> Tank1/2(F1)
  E1/1 -> Tank1/3(E1)
  T2/1 -> Tank2/5(T2)
  CT1/1 -> Tank1/1(CT1)
  MR2/1 -> Tank2/4(MR2)

== system c00003M_harness/M048 ==
  note: VALUES
      | ---------------------------------
      | ControlType = 1 | 2 | 3
      | FillTank = 0 | 1
      | EmptyTank = 0 | 1
      | ManualReference between 0 and 1
      | Tempreature between 0 and 100
      | EmergencyButton = 0 | 1
      | LiquidLevel between 0 and 1 (hmax)
  note: Inputs For Tank2
  note: NAMES
      | --------------------------------------------
      | CT1 = ControlType Tank 1
      | F1 = Fill Tank 1
      | E1 = Empty Tank 1
      | MR1 = Manual Reference Tank1
      | T1 = Temperature Tank 1
      | EB1 = Emergency Button Tank 1
      | LL1 = Liquid Level 1
  note: Inputs For Tank3
  note: Inputs For Tank1
  CT1 : Inport
  F1 : Inport  Port=2
  E1 : Inport  Port=3
  MR1 : Inport  Port=4
  T1 : Inport  Port=5
  EB1 : Inport  Port=6
  CT2 : Inport  Port=7
  F2 : Inport  Port=8
  E2 : Inport  Port=9
  MR2 : Inport  Port=10
  T2 : Inport  Port=11
  EB2 : Inport  Port=12
  Tank1 : Subsystem
  Tank2 : Subsystem
  LL1 : Outport
  LL2 : Outport  Port=2
  wires:
  EB1/1 -> Tank1/6(EB1)
  Tank2/1(LL2) -> LL2/1, Tank1/7(LL2)
  EB2/1 -> Tank2/6(EB2)
  CT2/1 -> Tank2/1(CT2)
  MR1/1 -> Tank1/4(MR1)
  T1/1 -> Tank1/5(T1)
  Tank1/1(LL1) -> LL1/1, Tank2/7(LL1)
  F2/1 -> Tank2/2(F2)
  E2/1 -> Tank2/3(E2)
  F1/1 -> Tank1/2(F1)
  E1/1 -> Tank1/3(E1)
  T2/1 -> Tank2/5(T2)
  CT1/1 -> Tank1/1(CT1)
  MR2/1 -> Tank2/4(MR2)

== system c00003M_harness/M049 ==
  note: VALUES
      | ---------------------------------
      | ControlType = 1 | 2 | 3
      | FillTank = 0 | 1
      | EmptyTank = 0 | 1
      | ManualReference between 0 and 1
      | Tempreature between 0 and 100
      | EmergencyButton = 0 | 1
      | LiquidLevel between 0 and 1 (hmax)
  note: Inputs For Tank2
  note: NAMES
      | --------------------------------------------
      | CT1 = ControlType Tank 1
      | F1 = Fill Tank 1
      | E1 = Empty Tank 1
      | MR1 = Manual Reference Tank1
      | T1 = Temperature Tank 1
      | EB1 = Emergency Button Tank 1
      | LL1 = Liquid Level 1
  note: Inputs For Tank3
  note: Inputs For Tank1
  CT1 : Inport
  F1 : Inport  Port=2
  E1 : Inport  Port=3
  MR1 : Inport  Port=4
  T1 : Inport  Port=5
  EB1 : Inport  Port=6
  CT2 : Inport  Port=7
  F2 : Inport  Port=8
  E2 : Inport  Port=9
  MR2 : Inport  Port=10
  T2 : Inport  Port=11
  EB2 : Inport  Port=12
  Tank1 : Subsystem
  Tank2 : Subsystem
  LL1 : Outport
  LL2 : Outport  Port=2
  wires:
  EB1/1 -> Tank1/6(EB1)
  Tank2/1(LL2) -> LL2/1, Tank1/7(LL2)
  EB2/1 -> Tank2/6(EB2)
  CT2/1 -> Tank2/1(CT2)
  MR1/1 -> Tank1/4(MR1)
  T1/1 -> Tank1/5(T1)
  Tank1/1(LL1) -> LL1/1, Tank2/7(LL1)
  F2/1 -> Tank2/2(F2)
  E2/1 -> Tank2/3(E2)
  F1/1 -> Tank1/2(F1)
  E1/1 -> Tank1/3(E1)
  T2/1 -> Tank2/5(T2)
  CT1/1 -> Tank1/1(CT1)
  MR2/1 -> Tank2/4(MR2)

== system c00003M_harness/M050 ==
  note: VALUES
      | ---------------------------------
      | ControlType = 1 | 2 | 3
      | FillTank = 0 | 1
      | EmptyTank = 0 | 1
      | ManualReference between 0 and 1
      | Tempreature between 0 and 100
      | EmergencyButton = 0 | 1
      | LiquidLevel between 0 and 1 (hmax)
  note: Inputs For Tank2
  note: NAMES
      | --------------------------------------------
      | CT1 = ControlType Tank 1
      | F1 = Fill Tank 1
      | E1 = Empty Tank 1
      | MR1 = Manual Reference Tank1
      | T1 = Temperature Tank 1
      | EB1 = Emergency Button Tank 1
      | LL1 = Liquid Level 1
  note: Inputs For Tank3
  note: Inputs For Tank1
  CT1 : Inport
  F1 : Inport  Port=2
  E1 : Inport  Port=3
  MR1 : Inport  Port=4
  T1 : Inport  Port=5
  EB1 : Inport  Port=6
  CT2 : Inport  Port=7
  F2 : Inport  Port=8
  E2 : Inport  Port=9
  MR2 : Inport  Port=10
  T2 : Inport  Port=11
  EB2 : Inport  Port=12
  Tank1 : Subsystem
  Tank2 : Subsystem
  LL1 : Outport
  LL2 : Outport  Port=2
  wires:
  EB1/1 -> Tank1/6(EB1)
  Tank2/1(LL2) -> LL2/1, Tank1/7(LL2)
  EB2/1 -> Tank2/6(EB2)
  CT2/1 -> Tank2/1(CT2)
  MR1/1 -> Tank1/4(MR1)
  T1/1 -> Tank1/5(T1)
  Tank1/1(LL1) -> LL1/1, Tank2/7(LL1)
  F2/1 -> Tank2/2(F2)
  E2/1 -> Tank2/3(E2)
  F1/1 -> Tank1/2(F1)
  E1/1 -> Tank1/3(E1)
  T2/1 -> Tank2/5(T2)
  CT1/1 -> Tank1/1(CT1)
  MR2/1 -> Tank2/4(MR2)

== system c00003M_harness/M051 ==
  note: VALUES
      | ---------------------------------
      | ControlType = 1 | 2 | 3
      | FillTank = 0 | 1
      | EmptyTank = 0 | 1
      | ManualReference between 0 and 1
      | Tempreature between 0 and 100
      | EmergencyButton = 0 | 1
      | LiquidLevel between 0 and 1 (hmax)
  note: Inputs For Tank2
  note: NAMES
      | --------------------------------------------
      | CT1 = ControlType Tank 1
      | F1 = Fill Tank 1
      | E1 = Empty Tank 1
      | MR1 = Manual Reference Tank1
      | T1 = Temperature Tank 1
      | EB1 = Emergency Button Tank 1
      | LL1 = Liquid Level 1
  note: Inputs For Tank3
  note: Inputs For Tank1
  CT1 : Inport
  F1 : Inport  Port=2
  E1 : Inport  Port=3
  MR1 : Inport  Port=4
  T1 : Inport  Port=5
  EB1 : Inport  Port=6
  CT2 : Inport  Port=7
  F2 : Inport  Port=8
  E2 : Inport  Port=9
  MR2 : Inport  Port=10
  T2 : Inport  Port=11
  EB2 : Inport  Port=12
  Tank1 : Subsystem
  Tank2 : Subsystem
  LL1 : Outport
  LL2 : Outport  Port=2
  wires:
  EB1/1 -> Tank1/6(EB1)
  Tank2/1(LL2) -> LL2/1, Tank1/7(LL2)
  EB2/1 -> Tank2/6(EB2)
  CT2/1 -> Tank2/1(CT2)
  MR1/1 -> Tank1/4(MR1)
  T1/1 -> Tank1/5(T1)
  Tank1/1(LL1) -> LL1/1, Tank2/7(LL1)
  F2/1 -> Tank2/2(F2)
  E2/1 -> Tank2/3(E2)
  F1/1 -> Tank1/2(F1)
  E1/1 -> Tank1/3(E1)
  T2/1 -> Tank2/5(T2)
  CT1/1 -> Tank1/1(CT1)
  MR2/1 -> Tank2/4(MR2)

== system c00003M_harness/M052 ==
  note: VALUES
      | ---------------------------------
      | ControlType = 1 | 2 | 3
      | FillTank = 0 | 1
      | EmptyTank = 0 | 1
      | ManualReference between 0 and 1
      | Tempreature between 0 and 100
      | EmergencyButton = 0 | 1
      | LiquidLevel between 0 and 1 (hmax)
  note: Inputs For Tank2
  note: NAMES
      | --------------------------------------------
      | CT1 = ControlType Tank 1
      | F1 = Fill Tank 1
      | E1 = Empty Tank 1
      | MR1 = Manual Reference Tank1
      | T1 = Temperature Tank 1
      | EB1 = Emergency Button Tank 1
      | LL1 = Liquid Level 1
  note: Inputs For Tank3
  note: Inputs For Tank1
  CT1 : Inport
  F1 : Inport  Port=2
  E1 : Inport  Port=3
  MR1 : Inport  Port=4
  T1 : Inport  Port=5
  EB1 : Inport  Port=6
  CT2 : Inport  Port=7
  F2 : Inport  Port=8
  E2 : Inport  Port=9
  MR2 : Inport  Port=10
  T2 : Inport  Port=11
  EB2 : Inport  Port=12
  Tank1 : Subsystem
  Tank2 : Subsystem
  LL1 : Outport
  LL2 : Outport  Port=2
  wires:
  EB1/1 -> Tank1/6(EB1)
  Tank2/1(LL2) -> LL2/1, Tank1/7(LL2)
  EB2/1 -> Tank2/6(EB2)
  CT2/1 -> Tank2/1(CT2)
  MR1/1 -> Tank1/4(MR1)
  T1/1 -> Tank1/5(T1)
  Tank1/1(LL1) -> LL1/1, Tank2/7(LL1)
  F2/1 -> Tank2/2(F2)
  E2/1 -> Tank2/3(E2)
  F1/1 -> Tank1/2(F1)
  E1/1 -> Tank1/3(E1)
  T2/1 -> Tank2/5(T2)
  CT1/1 -> Tank1/1(CT1)
  MR2/1 -> Tank2/4(MR2)

== system c00003M_harness/M053 ==
  note: VALUES
      | ---------------------------------
      | ControlType = 1 | 2 | 3
      | FillTank = 0 | 1
      | EmptyTank = 0 | 1
      | ManualReference between 0 and 1
      | Tempreature between 0 and 100
      | EmergencyButton = 0 | 1
      | LiquidLevel between 0 and 1 (hmax)
  note: Inputs For Tank2
  note: NAMES
      | --------------------------------------------
      | CT1 = ControlType Tank 1
      | F1 = Fill Tank 1
      | E1 = Empty Tank 1
      | MR1 = Manual Reference Tank1
      | T1 = Temperature Tank 1
      | EB1 = Emergency Button Tank 1
      | LL1 = Liquid Level 1
  note: Inputs For Tank3
  note: Inputs For Tank1
  CT1 : Inport
  F1 : Inport  Port=2
  E1 : Inport  Port=3
  MR1 : Inport  Port=4
  T1 : Inport  Port=5
  EB1 : Inport  Port=6
  CT2 : Inport  Port=7
  F2 : Inport  Port=8
  E2 : Inport  Port=9
  MR2 : Inport  Port=10
  T2 : Inport  Port=11
  EB2 : Inport  Port=12
  Tank1 : Subsystem
  Tank2 : Subsystem
  LL1 : Outport
  LL2 : Outport  Port=2
  wires:
  EB1/1 -> Tank1/6(EB1)
  Tank2/1(LL2) -> LL2/1, Tank1/7(LL2)
  EB2/1 -> Tank2/6(EB2)
  CT2/1 -> Tank2/1(CT2)
  MR1/1 -> Tank1/4(MR1)
  T1/1 -> Tank1/5(T1)
  Tank1/1(LL1) -> LL1/1, Tank2/7(LL1)
  F2/1 -> Tank2/2(F2)
  E2/1 -> Tank2/3(E2)
  F1/1 -> Tank1/2(F1)
  E1/1 -> Tank1/3(E1)
  T2/1 -> Tank2/5(T2)
  CT1/1 -> Tank1/1(CT1)
  MR2/1 -> Tank2/4(MR2)

== system c00003M_harness/M054 ==
  note: VALUES
      | ---------------------------------
      | ControlType = 1 | 2 | 3
      | FillTank = 0 | 1
      | EmptyTank = 0 | 1
      | ManualReference between 0 and 1
      | Tempreature between 0 and 100
      | EmergencyButton = 0 | 1
      | LiquidLevel between 0 and 1 (hmax)
  note: Inputs For Tank2
  note: NAMES
      | --------------------------------------------
      | CT1 = ControlType Tank 1
      | F1 = Fill Tank 1
      | E1 = Empty Tank 1
      | MR1 = Manual Reference Tank1
      | T1 = Temperature Tank 1
      | EB1 = Emergency Button Tank 1
      | LL1 = Liquid Level 1
  note: Inputs For Tank3
  note: Inputs For Tank1
  CT1 : Inport
  F1 : Inport  Port=2
  E1 : Inport  Port=3
  MR1 : Inport  Port=4
  T1 : Inport  Port=5
  EB1 : Inport  Port=6
  CT2 : Inport  Port=7
  F2 : Inport  Port=8
  E2 : Inport  Port=9
  MR2 : Inport  Port=10
  T2 : Inport  Port=11
  EB2 : Inport  Port=12
  Tank1 : Subsystem
  Tank2 : Subsystem
  LL1 : Outport
  LL2 : Outport  Port=2
  wires:
  EB1/1 -> Tank1/6(EB1)
  Tank2/1(LL2) -> LL2/1, Tank1/7(LL2)
  EB2/1 -> Tank2/6(EB2)
  CT2/1 -> Tank2/1(CT2)
  MR1/1 -> Tank1/4(MR1)
  T1/1 -> Tank1/5(T1)
  Tank1/1(LL1) -> LL1/1, Tank2/7(LL1)
  F2/1 -> Tank2/2(F2)
  E2/1 -> Tank2/3(E2)
  F1/1 -> Tank1/2(F1)
  E1/1 -> Tank1/3(E1)
  T2/1 -> Tank2/5(T2)
  CT1/1 -> Tank1/1(CT1)
  MR2/1 -> Tank2/4(MR2)

== system c00003M_harness/M055 ==
  note: VALUES
      | ---------------------------------
      | ControlType = 1 | 2 | 3
      | FillTank = 0 | 1
      | EmptyTank = 0 | 1
      | ManualReference between 0 and 1
      | Tempreature between 0 and 100
      | EmergencyButton = 0 | 1
      | LiquidLevel between 0 and 1 (hmax)
  note: Inputs For Tank2
  note: NAMES
      | --------------------------------------------
      | CT1 = ControlType Tank 1
      | F1 = Fill Tank 1
      | E1 = Empty Tank 1
      | MR1 = Manual Reference Tank1
      | T1 = Temperature Tank 1
      | EB1 = Emergency Button Tank 1
      | LL1 = Liquid Level 1
  note: Inputs For Tank3
  note: Inputs For Tank1
  CT1 : Inport
  F1 : Inport  Port=2
  E1 : Inport  Port=3
  MR1 : Inport  Port=4
  T1 : Inport  Port=5
  EB1 : Inport  Port=6
  CT2 : Inport  Port=7
  F2 : Inport  Port=8
  E2 : Inport  Port=9
  MR2 : Inport  Port=10
  T2 : Inport  Port=11
  EB2 : Inport  Port=12
  Tank1 : Subsystem
  Tank2 : Subsystem
  LL1 : Outport
  LL2 : Outport  Port=2
  wires:
  EB1/1 -> Tank1/6(EB1)
  Tank2/1(LL2) -> LL2/1, Tank1/7(LL2)
  EB2/1 -> Tank2/6(EB2)
  CT2/1 -> Tank2/1(CT2)
  MR1/1 -> Tank1/4(MR1)
  T1/1 -> Tank1/5(T1)
  Tank1/1(LL1) -> LL1/1, Tank2/7(LL1)
  F2/1 -> Tank2/2(F2)
  E2/1 -> Tank2/3(E2)
  F1/1 -> Tank1/2(F1)
  E1/1 -> Tank1/3(E1)
  T2/1 -> Tank2/5(T2)
  CT1/1 -> Tank1/1(CT1)
  MR2/1 -> Tank2/4(MR2)

== system c00003M_harness/M056 ==
  note: VALUES
      | ---------------------------------
      | ControlType = 1 | 2 | 3
      | FillTank = 0 | 1
      | EmptyTank = 0 | 1
      | ManualReference between 0 and 1
      | Tempreature between 0 and 100
      | EmergencyButton = 0 | 1
      | LiquidLevel between 0 and 1 (hmax)
  note: Inputs For Tank2
  note: NAMES
      | --------------------------------------------
      | CT1 = ControlType Tank 1
      | F1 = Fill Tank 1
      | E1 = Empty Tank 1
      | MR1 = Manual Reference Tank1
      | T1 = Temperature Tank 1
      | EB1 = Emergency Button Tank 1
      | LL1 = Liquid Level 1
  note: Inputs For Tank3
  note: Inputs For Tank1
  CT1 : Inport
  F1 : Inport  Port=2
  E1 : Inport  Port=3
  MR1 : Inport  Port=4
  T1 : Inport  Port=5
  EB1 : Inport  Port=6
  CT2 : Inport  Port=7
  F2 : Inport  Port=8
  E2 : Inport  Port=9
  MR2 : Inport  Port=10
  T2 : Inport  Port=11
  EB2 : Inport  Port=12
  Tank1 : Subsystem
  Tank2 : Subsystem
  LL1 : Outport
  LL2 : Outport  Port=2
  wires:
  EB1/1 -> Tank1/6(EB1)
  Tank2/1(LL2) -> LL2/1, Tank1/7(LL2)
  EB2/1 -> Tank2/6(EB2)
  CT2/1 -> Tank2/1(CT2)
  MR1/1 -> Tank1/4(MR1)
  T1/1 -> Tank1/5(T1)
  Tank1/1(LL1) -> LL1/1, Tank2/7(LL1)
  F2/1 -> Tank2/2(F2)
  E2/1 -> Tank2/3(E2)
  F1/1 -> Tank1/2(F1)
  E1/1 -> Tank1/3(E1)
  T2/1 -> Tank2/5(T2)
  CT1/1 -> Tank1/1(CT1)
  MR2/1 -> Tank2/4(MR2)

== system c00003M_harness/M058 ==
  note: VALUES
      | ---------------------------------
      | ControlType = 1 | 2 | 3
      | FillTank = 0 | 1
      | EmptyTank = 0 | 1
      | ManualReference between 0 and 1
      | Tempreature between 0 and 100
      | EmergencyButton = 0 | 1
      | LiquidLevel between 0 and 1 (hmax)
  note: Inputs For Tank2
  note: NAMES
      | --------------------------------------------
      | CT1 = ControlType Tank 1
      | F1 = Fill Tank 1
      | E1 = Empty Tank 1
      | MR1 = Manual Reference Tank1
      | T1 = Temperature Tank 1
      | EB1 = Emergency Button Tank 1
      | LL1 = Liquid Level 1
  note: Inputs For Tank3
  note: Inputs For Tank1
  CT1 : Inport
  F1 : Inport  Port=2
  E1 : Inport  Port=3
  MR1 : Inport  Port=4
  T1 : Inport  Port=5
  EB1 : Inport  Port=6
  CT2 : Inport  Port=7
  F2 : Inport  Port=8
  E2 : Inport  Port=9
  MR2 : Inport  Port=10
  T2 : Inport  Port=11
  EB2 : Inport  Port=12
  Tank1 : Subsystem
  Tank2 : Subsystem
  LL1 : Outport
  LL2 : Outport  Port=2
  wires:
  EB1/1 -> Tank1/6(EB1)
  Tank2/1(LL2) -> LL2/1, Tank1/7(LL2)
  EB2/1 -> Tank2/6(EB2)
  CT2/1 -> Tank2/1(CT2)
  MR1/1 -> Tank1/4(MR1)
  T1/1 -> Tank1/5(T1)
  Tank1/1(LL1) -> LL1/1, Tank2/7(LL1)
  F2/1 -> Tank2/2(F2)
  E2/1 -> Tank2/3(E2)
  F1/1 -> Tank1/2(F1)
  E1/1 -> Tank1/3(E1)
  T2/1 -> Tank2/5(T2)
  CT1/1 -> Tank1/1(CT1)
  MR2/1 -> Tank2/4(MR2)

== system c00003M_harness/M059 ==
  note: VALUES
      | ---------------------------------
      | ControlType = 1 | 2 | 3
      | FillTank = 0 | 1
      | EmptyTank = 0 | 1
      | ManualReference between 0 and 1
      | Tempreature between 0 and 100
      | EmergencyButton = 0 | 1
      | LiquidLevel between 0 and 1 (hmax)
  note: Inputs For Tank2
  note: NAMES
      | --------------------------------------------
      | CT1 = ControlType Tank 1
      | F1 = Fill Tank 1
      | E1 = Empty Tank 1
      | MR1 = Manual Reference Tank1
      | T1 = Temperature Tank 1
      | EB1 = Emergency Button Tank 1
      | LL1 = Liquid Level 1
  note: Inputs For Tank3
  note: Inputs For Tank1
  CT1 : Inport
  F1 : Inport  Port=2
  E1 : Inport  Port=3
  MR1 : Inport  Port=4
  T1 : Inport  Port=5
  EB1 : Inport  Port=6
  CT2 : Inport  Port=7
  F2 : Inport  Port=8
  E2 : Inport  Port=9
  MR2 : Inport  Port=10
  T2 : Inport  Port=11
  EB2 : Inport  Port=12
  Tank1 : Subsystem
  Tank2 : Subsystem
  LL1 : Outport
  LL2 : Outport  Port=2
  wires:
  EB1/1 -> Tank1/6(EB1)
  Tank2/1(LL2) -> LL2/1, Tank1/7(LL2)
  EB2/1 -> Tank2/6(EB2)
  CT2/1 -> Tank2/1(CT2)
  MR1/1 -> Tank1/4(MR1)
  T1/1 -> Tank1/5(T1)
  Tank1/1(LL1) -> LL1/1, Tank2/7(LL1)
  F2/1 -> Tank2/2(F2)
  E2/1 -> Tank2/3(E2)
  F1/1 -> Tank1/2(F1)
  E1/1 -> Tank1/3(E1)
  T2/1 -> Tank2/5(T2)
  CT1/1 -> Tank1/1(CT1)
  MR2/1 -> Tank2/4(MR2)

== system c00003M_harness/M060 ==
  note: VALUES
      | ---------------------------------
      | ControlType = 1 | 2 | 3
      | FillTank = 0 | 1
      | EmptyTank = 0 | 1
      | ManualReference between 0 and 1
      | Tempreature between 0 and 100
      | EmergencyButton = 0 | 1
      | LiquidLevel between 0 and 1 (hmax)
  note: Inputs For Tank2
  note: NAMES
      | --------------------------------------------
      | CT1 = ControlType Tank 1
      | F1 = Fill Tank 1
      | E1 = Empty Tank 1
      | MR1 = Manual Reference Tank1
      | T1 = Temperature Tank 1
      | EB1 = Emergency Button Tank 1
      | LL1 = Liquid Level 1
  note: Inputs For Tank3
  note: Inputs For Tank1
  CT1 : Inport
  F1 : Inport  Port=2
  E1 : Inport  Port=3
  MR1 : Inport  Port=4
  T1 : Inport  Port=5
  EB1 : Inport  Port=6
  CT2 : Inport  Port=7
  F2 : Inport  Port=8
  E2 : Inport  Port=9
  MR2 : Inport  Port=10
  T2 : Inport  Port=11
  EB2 : Inport  Port=12
  Tank1 : Subsystem
  Tank2 : Subsystem
  LL1 : Outport
  LL2 : Outport  Port=2
  wires:
  EB1/1 -> Tank1/6(EB1)
  Tank2/1(LL2) -> LL2/1, Tank1/7(LL2)
  EB2/1 -> Tank2/6(EB2)
  CT2/1 -> Tank2/1(CT2)
  MR1/1 -> Tank1/4(MR1)
  T1/1 -> Tank1/5(T1)
  Tank1/1(LL1) -> LL1/1, Tank2/7(LL1)
  F2/1 -> Tank2/2(F2)
  E2/1 -> Tank2/3(E2)
  F1/1 -> Tank1/2(F1)
  E1/1 -> Tank1/3(E1)
  T2/1 -> Tank2/5(T2)
  CT1/1 -> Tank1/1(CT1)
  MR2/1 -> Tank2/4(MR2)

== system c00003M_harness/M061 ==
  note: VALUES
      | ---------------------------------
      | ControlType = 1 | 2 | 3
      | FillTank = 0 | 1
      | EmptyTank = 0 | 1
      | ManualReference between 0 and 1
      | Tempreature between 0 and 100
      | EmergencyButton = 0 | 1
      | LiquidLevel between 0 and 1 (hmax)
  note: Inputs For Tank2
  note: NAMES
      | --------------------------------------------
      | CT1 = ControlType Tank 1
      | F1 = Fill Tank 1
      | E1 = Empty Tank 1
      | MR1 = Manual Reference Tank1
      | T1 = Temperature Tank 1
      | EB1 = Emergency Button Tank 1
      | LL1 = Liquid Level 1
  note: Inputs For Tank3
  note: Inputs For Tank1
  CT1 : Inport
  F1 : Inport  Port=2
  E1 : Inport  Port=3
  MR1 : Inport  Port=4
  T1 : Inport  Port=5
  EB1 : Inport  Port=6
  CT2 : Inport  Port=7
  F2 : Inport  Port=8
  E2 : Inport  Port=9
  MR2 : Inport  Port=10
  T2 : Inport  Port=11
  EB2 : Inport  Port=12
  Tank1 : Subsystem
  Tank2 : Subsystem
  LL1 : Outport
  LL2 : Outport  Port=2
  wires:
  EB1/1 -> Tank1/6(EB1)
  Tank2/1(LL2) -> LL2/1, Tank1/7(LL2)
  EB2/1 -> Tank2/6(EB2)
  CT2/1 -> Tank2/1(CT2)
  MR1/1 -> Tank1/4(MR1)
  T1/1 -> Tank1/5(T1)
  Tank1/1(LL1) -> LL1/1, Tank2/7(LL1)
  F2/1 -> Tank2/2(F2)
  E2/1 -> Tank2/3(E2)
  F1/1 -> Tank1/2(F1)
  E1/1 -> Tank1/3(E1)
  T2/1 -> Tank2/5(T2)
  CT1/1 -> Tank1/1(CT1)
  MR2/1 -> Tank2/4(MR2)
